simulink model "OneDegreeFreedom_Model"  (R2019a)
settings: Solver=VariableStepAuto  StartTime=0.0  StopTime=10.0  RelTol=1e-3
undefined symbols (not defined in the file): C_s, K_s, m_s
settings Model: Creator=ansar  LastModifiedBy=ansar

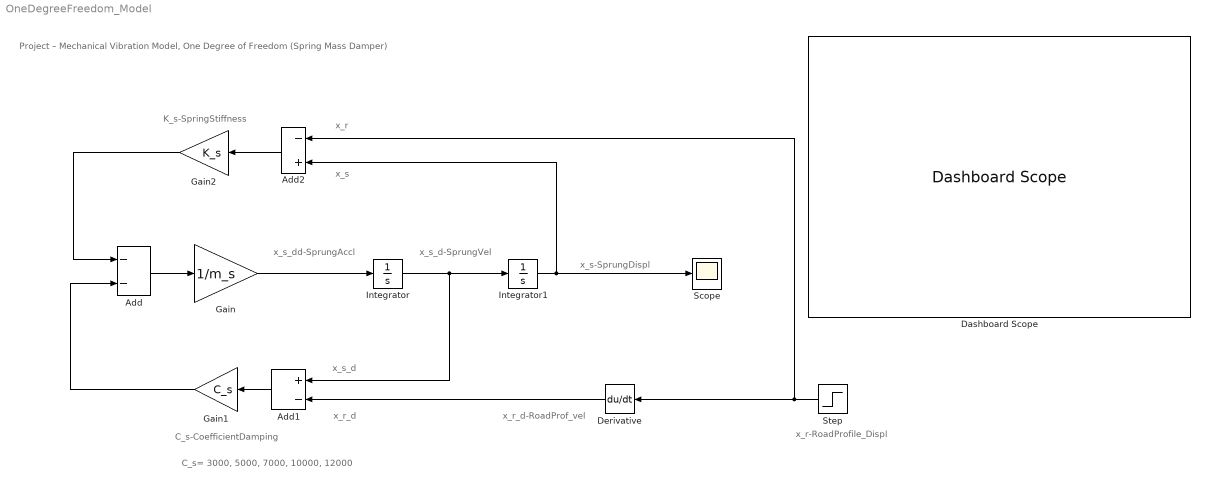
== system OneDegreeFreedom_Model ==
  note: C_s-CoefficientDamping
  note: K_s-SpringStiffness
  note: C_s= 3000, 5000, 7000, 10000, 12000
  note: x_r
  note: x_s
  note: x_s_d
  note: x_r_d
  note: x_r_d-RoadProf_vel
  note: x_r-RoadProfile_Displ
  note: x_s-SprungDispl
  note: x_s_d-SprungVel
  note: x_s_dd-SprungAccl
  note: Project – Mechanical Vibration Model, One Degree of Freedom (Spring Mass Damper)
  Add : Sum  Inputs=--
  Add1 : Sum  Inputs=+-
  Add2 : Sum  Inputs=-+
  Dashboard Scope : DashboardScope
  Derivative : Derivative
  Gain : Gain  Gain=1/m_s
  Gain1 : Gain  Gain=C_s
  Gain2 : Gain  Gain=K_s
  Integrator : Integrator
  Integrator1 : Integrator
  Scope : Scope
  Step : Step  After=10  SampleTime=0
  wires:
  Add/1 -> Gain/1
  Gain1/1 -> Add/2
  Add1/1 -> Gain1/1
  Derivative/1 -> Add1/2
  Gain/1 -> Integrator/1
  Gain2/1 -> Add/1
  Add2/1 -> Gain2/1
  Integrator/1 -> Add1/1, Integrator1/1
  Integrator1/1 -> Scope/1, Add2/2
  Step/1 -> Add2/1, Derivative/1
